simulink model "lapSim"  (R2026a)
settings: Solver=VariableStepAuto
settings Model: Creator=axelg  LastModifiedBy=axelg

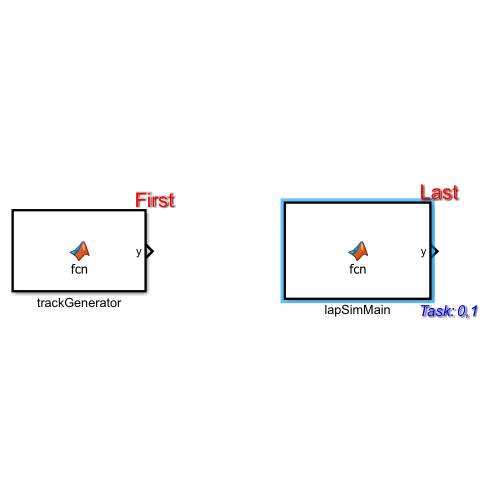
[thumbnail: Simulink's stored preview of the top-level diagram]
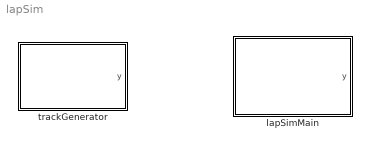
== system lapSim ==
  lapSimMain : MATLAB Function  ExecutionOrder=Last  TreatAsAtomicUnit=on
  trackGenerator : MATLAB Function  ExecutionOrder=First  TreatAsAtomicUnit=on

== matlab function lapSim/lapSimMain ==
  data: y output
function y = fcn()
    coder.extrinsic('evalin')
    persistent done
    if isempty(done)
        done = false;
    end

    y = 0;
    
    if ~done
        evalin('base', 'LapSimMain')
        done = true;
    end
end

== matlab function lapSim/trackGenerator ==
  data: y output
function y = fcn()
    coder.extrinsic('trackGenerator');
    persistent done
    if isempty(done)
        done = false;
    end


    y = 0;
    hold off;
    if ~done
        trackGenerator('gps_comp.csv');
        done = true;
    end
end
